simulink model "newproject_simulation"  (R2020b)
settings: Solver=VariableStepAuto  StartTime=0.0  StopTime=1  RelTol=1e-3
libraries: powerlib x22
settings Model: Creator=mrsan  LastModifiedBy=mrsan
settings SolverCC: ZeroCrossAlgorithm=Adaptive
settings DebuggingCC: MaskedZcDiagnostic=none  IgnoredZcDiagnostic=none

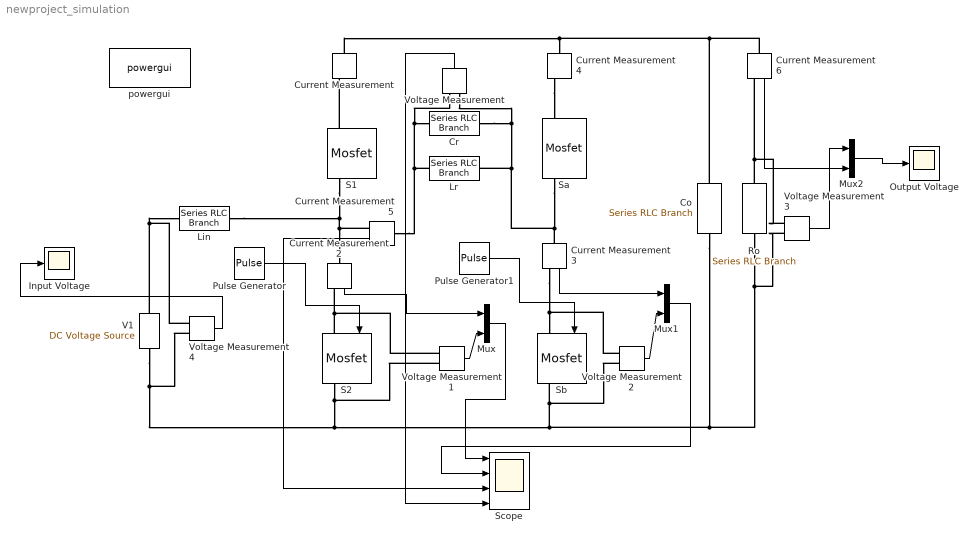
== system newproject_simulation ==
  Co : powerlib/Elements/Series RLC Branch  LConnTagsString=__new0  RConnTagsString=__new0  BranchType=C  Resistance=1  Inductance=1e-3  SetiL0=off  InitialCurrent=0  Capacitance=0.000470  Setx0=off  InitialVoltage=0  Measurements=None
  Cr : powerlib/Elements/Series RLC Branch  LConnTagsString=__new0  RConnTagsString=__new0  BranchType=C  Resistance=1  Inductance=1e-3  SetiL0=off  InitialCurrent=0  Capacitance=0.000000010  Setx0=off  InitialVoltage=0  Measurements=None
  Current Measurement{,2..6} (6 alike) : powerlib/Measurements/Current Measurement  PhasorSimulation=off  OutputType=Complex  PSBequivalent=0
  Input Voltage : Scope
  Lin : powerlib/Elements/Series RLC Branch  LConnTagsString=__new0  RConnTagsString=__new0  BranchType=L  Resistance=1  Inductance=0.0001  SetiL0=off  InitialCurrent=0  Capacitance=1e-6  Setx0=off  InitialVoltage=0  Measurements=None
  Lr : powerlib/Elements/Series RLC Branch  LConnTagsString=__new0  RConnTagsString=__new0  BranchType=L  Resistance=1  Inductance=0.000002  SetiL0=off  InitialCurrent=0  Capacitance=1e-6  Setx0=off  InitialVoltage=0  Measurements=None
  Mux : Mux  Inputs=2
  Mux1 : Mux  Inputs=2
  Mux2 : Mux  Inputs=2
  Output Voltage : Scope
  Pulse Generator : DiscretePulseGenerator  PulseType=Time based  Period=1/30000  PulseWidth=50
  Pulse Generator1 : DiscretePulseGenerator  PulseType=Time based  Period=1/30000  PulseWidth=10
  Ro : powerlib/Elements/Series RLC Branch  LConnTagsString=__new0  RConnTagsString=__new0  BranchType=R  Resistance=14.4  Inductance=1e-3  SetiL0=off  InitialCurrent=0  Capacitance=1e-6  Setx0=off  InitialVoltage=0  Measurements=None
  S1 : powerlib/Power Electronics/Mosfet  Ron=0.1  Lon=0  Rd=0.01  Vfd=0  IC=0  Rs=1e5  Cs=inf  Measurements=on
  S2 : powerlib/Power Electronics/Mosfet  Ron=0.1  Lon=0  Rd=0.01  Vfd=0  IC=0  Rs=1e5  Cs=inf  Measurements=on
  Sa : powerlib/Power Electronics/Mosfet  Ron=0.1  Lon=0  Rd=0.01  Vfd=0  IC=0  Rs=1e5  Cs=inf  Measurements=on
  Sb : powerlib/Power Electronics/Mosfet  Ron=0.1  Lon=0  Rd=0.01  Vfd=0  IC=0  Rs=1e5  Cs=inf  Measurements=on
  Scope : Scope  NumInputPorts=4
  V1 : powerlib/Electrical Sources/DC Voltage Source  Amplitude=200  Measurements=None
  Voltage Measurement{,1..4} (5 alike) : powerlib/Measurements/Voltage Measurement  PhasorSimulation=off  OutputType=Complex  PSBequivalent=0
  powergui : powerlib/powergui  Priority=1  SimulationMode=Continuous  SampleTime=50e-6  frequency=60  Iterations=50  frequencyindice=0  Pbase=100e6  ErrMax=1e-4  UnitsV=kV  UnitsW=MW  buscounter=0  FunctionMessages=off  echomessages=off  EnableUseOfTLC=off  CurrentSourceSwitches=off  DisableSnubberDevices=off  DisableRonSwitches=off  DisableVfSwitches=off  DisplayEquations=off  AutomaticDiscreteSolvers=off  SolverType=Tustin/Backward Euler (TBE)  Interpol=off  ExternalGateDelay=off  methode=off  Ts=100  x0status=blocks  SPID=on  SwTol=0  HookPort=off  NonlinearTolerance=1e-4  nMaxIteration=100  ContinueOnMaxIteration=off  RestoreLinks=warning  ResistiveCurrentMeasurement=off  Frange=[0:2:500]  Ylog=off  Xlog=on  ShowGrid=off  save=off  variable=ZData  structure=0  ZoomFFT=off  StartTime=0.0  cycles=1  DisplayStyle=1  fundamental=60  FreqAxis=off  MaxFrequency=1000  frequencyindicesteady=1  RmsSteady=1  display=off
  wires:
  Voltage Measurement1/1 -> Mux/2
  Voltage Measurement2/1 -> Mux1/2
  Current Measurement3/1 -> Mux1/1
  Voltage Measurement/1 -> Scope/4
  Mux1/1 -> Scope/2
  Current Measurement2/1 -> Mux/1
  Current Measurement6/1 -> Mux2/2
  Voltage Measurement3/1 -> Mux2/1
  Mux2/1 -> Output Voltage/1
  Current Measurement5/1 -> Scope/3
  Mux/1 -> Scope/1
  Voltage Measurement4/1 -> Input Voltage/1
  Pulse Generator/1 -> S2/1
  Pulse Generator1/1 -> Sb/1
  connections:
  S1/LConn1 -- Current Measurement/RConn1
  S1/RConn1 -- Current Measurement5/RConn1 -- Current Measurement2/LConn1 -- Lin/RConn1
  S2/LConn1 -- Current Measurement2/RConn1 -- Voltage Measurement1/LConn1
  Current Measurement3/RConn1 -- Voltage Measurement2/LConn1 -- Sb/LConn1
  Current Measurement4/RConn1 -- Sa/LConn1
  Current Measurement/LConn1 -- Co/LConn1 -- Current Measurement6/LConn1 -- Current Measurement4/LConn1
  S2/RConn1 -- Voltage Measurement1/LConn2 -- V1/LConn1 -- Voltage Measurement4/LConn2 -- Ro/RConn1 -- Voltage Measurement3/LConn2 -- Co/RConn1 -- Voltage Measurement2/LConn2 -- Sb/RConn1
  V1/RConn1 -- Voltage Measurement4/LConn1 -- Lin/LConn1
  Lr/LConn1 -- Current Measurement5/LConn1 -- Voltage Measurement/LConn1 -- Cr/LConn1
  Cr/RConn1 -- Lr/RConn1 -- Sa/RConn1 -- Current Measurement3/LConn1 -- Voltage Measurement/LConn2
  Ro/LConn1 -- Current Measurement6/RConn1 -- Voltage Measurement3/LConn1
